simulink model "UPSControl"  (R2025b)
settings: Solver=VariableStepAuto  StartTime=0.0  StopTime=10  FixedStep=Ts  RelTol=1e-3
PostLoadFcn:
  | DataCenterParam;
values from neighbouring files (symbols this model uses):
  generator = struct    [GeneratorParam.m]
  lineInductance = 1e-6    (= 1e-06)    [DataCenterParam.m]    (also in GridParam.m)
  lineResistance = 1e-3    (= 0.001)    [DataCenterParam.m]    (also in GridParam.m)
  loadPower = 5e6    (= 5000000)    [DataCenterParam.m]    (also in LVRT.m; RedundancyAnalysis.m = 10000000)
  machine = struct    [GeneratorParam.m]
  powerTau = 0.005    [DataCenterParam.m]
  Ts = 5e-5    (= 5e-05)    [DataCenterParam.m]    (also in GeneratorParam.m)
  utilizationFactor = 0.45    [DataCenterParam.m]    (also in RedundancyAnalysis.m)
undefined symbols (not defined in the file or in its folder): breaker, ctLimitDelayTime, DiscIntNeverNeededParam, ee_sli_rtmsupport, gcbh, grid, rack, ups
libraries: nesl_utility x96, fl_lib x96, eeGeneralControl x84, ee_lib x80, simulink x68, eeTransforms x30, nesl_utility_internal x16, eeSinusoidalMeasurementV2 x13, slpidlib x12, simulink_extras x12, datacenter_lib x5, batteryecm_lib x4
(part 1 of 13)
settings Model: SimulationMode=accelerator  Creator=skota  LastModifiedBy=vikrants
settings SolverCC: ZeroCrossAlgorithm=Adaptive
settings DataIOCC: SaveOutput=off  DSMLogging=off  StreamToWks=off  SaveTime=off  ReturnWorkspaceOutputs=off
settings SimscapeCC: SimscapeCompileComponentReuse=on

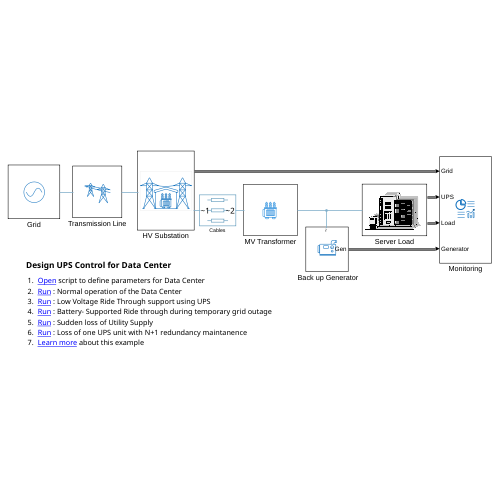
[thumbnail: Simulink's stored preview of the top-level diagram]
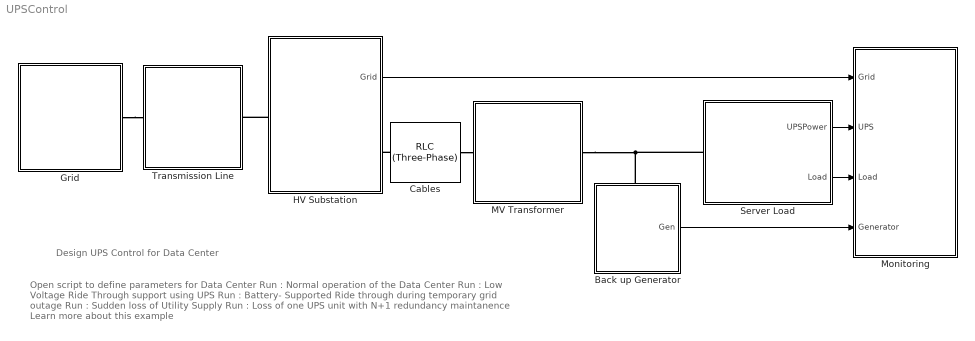
== system UPSControl ==
  note: Design UPS Control for Data Center
  note: Open script to define parameters for Data Center
      | Run : Normal operation of the Data Center
      | Run : Low Voltage Ride Through support using UPS
      | Run : Battery- Supported Ride through during temporary grid outage
      | Run : Sudden loss of Utility Supply
      | Run : Loss of one UPS unit with N+1 redundancy maintanence
      | Learn more about this example
  " Back up Generator" : Subsystem
      settings: PortSchema="{\"entries\":[{\"content\":{\"sides\":[{\"content\":{},\"type\":\"ConnectorPlacement.EquallySpacedRectSide\",\"uuid\":\"0e4bb094-5f01-4715-b678-e6b326bbface\"},{\"content\":{\"connectorIds\":[\"Out1\"],\"side\":\"RIGHT\"},\"type\":\"ConnectorPlacement.EquallySpacedRectSide\",\"uuid\":\"0cb60177-20db-48f9-a9cc-070daf12251a\"},{\"content\":{\"connectorIds\":[\"LConn1\"],\"side\":\"TOP\"},\"type\":\"ConnectorPlacement.EquallySpacedRectSide\",\"uuid\":\"205cef4a-01a9-469e-ade5-58cd4fb704d4\"},{\"content\":{\"side\":\"BOTTOM\"},\"type\":\"ConnectorPlacement.EquallySpacedRectSide\",\"uuid\":\"006e0ade-b558-4494-a2f0-eb5d5c15551c\"}]},\"type\":\"ConnectorPlacement.EquallySpacedConnector\",\"uuid\":\"9a4799c2-8742-4ae9-b78d-c2acced826f3\"}],\"packageUris\":[\"http://schema.mathworks.com/mf0/Connector/R2020b\"],\"version\":\"1.0\"}"
  Cables : ee_lib/Passive/RLC Assemblies/RLC (Three-Phase)  port_option=ee.enum.threePhasePort.composite  component_structure=ee.enum.rlc.structure.SeriesRL  R=lineResistance Ohm  L=lineInductance H  C=1e-6 F  R_parasitic=0 Ohm  G_parasitic=0 1/Ohm  IL_specify=on  IL_priority=None  IL=[0, 0, 0] A  IL_nominal_specify=off  IL_nominal_value=1  IL_nominal_unit=A  VC_specify=off  VC_priority=High  VC=[0, 0, 0] V  VC_nominal_specify=off  VC_nominal_value=1  VC_nominal_unit=V
      settings: InternalSimscapePortConfiguration="{\"Bottom\":[],\"Left\":[{\"id\":\"N1\",\"label\":\"~1\",\"type\":\"foundation.electrical.three_phase\"}],\"Right\":[{\"id\":\"N2\",\"label\":\"~2\",\"type\":\"foundation.electrical.three_phase\"}],\"Top\":[]}"
  Grid : Subsystem
  HV Substation : Subsystem
  MV Transformer : Subsystem
  Monitoring : Subsystem
  Server Load : Subsystem
      mask Display: image('datacenter.png');
  Transmission Line : Subsystem
  wires:
  Server Load/1(UPSPower) -> Monitoring/2(UPS)
  HV Substation/1(Grid) -> Monitoring/1(Grid)
  " Back up Generator"/1(Gen) -> Monitoring/4(Generator)
  Server Load/2(Load) -> Monitoring/3(Load)
  connections:
  Cables/LConn1 -- HV Substation/RConn1
  Cables/RConn1 -- MV Transformer/LConn1
  MV Transformer/RConn1 -- Server Load/LConn1 -- " Back up Generator"/LConn1
  HV Substation/LConn1 -- Transmission Line/LConn1
  Grid/LConn1 -- Transmission Line/RConn1

== system UPSControl/ Back up Generator ==
  note: Circuit breaker
  Brk Signal : Step  Time=breaker.generator  Before=1  After=0  SampleTime=0
  Cables : ee_lib/Passive/RLC Assemblies/RLC (Three-Phase)  port_option=ee.enum.threePhasePort.composite  component_structure=ee.enum.rlc.structure.SeriesRL  R=1e-3 Ohm  L=1e-5 H  C=1e-6 F  R_parasitic=0 Ohm  G_parasitic=0 1/Ohm  IL_specify=on  IL_priority=None  IL=[0, 0, 0] A  IL_nominal_specify=off  IL_nominal_value=1  IL_nominal_unit=A  VC_specify=off  VC_priority=High  VC=[0, 0, 0] V  VC_nominal_specify=off  VC_nominal_value=1  VC_nominal_unit=V
      settings: InternalSimscapePortConfiguration="{\"Bottom\":[],\"Left\":[{\"id\":\"N1\",\"label\":\"~1\",\"type\":\"foundation.electrical.three_phase\"}],\"Right\":[{\"id\":\"N2\",\"label\":\"~2\",\"type\":\"foundation.electrical.three_phase\"}],\"Top\":[]}"
  Constant : Constant  Value=0
  Generator Set : Subsystem  Variant=on  VariantControlMode=label  LabelModeActiveChoice=Detailed  mask(Generator){fidelity=Detailed, genRating=generator.rating, Vac=generator.Vac, frequency=generator.frequency, polePairs=generator.polePairs, pu_speed_reference=machine.speedReference, droop_percentage=machine.droop, pu_load_reference_setpoint=machine.loadReference, T_G=machine.timeConstandGovernor, T_CH=machine.timeConstantPrimeMover, base_torque=machine.baseTorque, pu_torque0=machine.initialTorque}
      mask prompts: fidelity "Modeling Option"; genRating "Generator Rating (kW)"; Vac "Rated AC side voltage (phase-phase RMS) (V)"; frequency "Rated electrical frequency at AC side (Hz)"; polePairs "Number of pole pairs"; pu_speed_reference "Speed reference, (pu)"; droop_percentage "Percentage droop, (%)"; pu_load_reference_setpoint "Load reference setpoint, (pu)"; T_G "Time constant of governor, (s)"; T_CH "Time constant of main inlet volumes and steam chest, (s)"; base_torque "Base torque, (N*m)"; pu_torque0 "Initial torque, (pu)"
      mask help:
      | This block models a Generator. The detailed variant models AVR, Exciter, Prime mover, and Governer. The simplified variant is based on load torque and a constant field circuit current. Select simplified mode for faster simulation using fixed efficiency and rated power.
      |
      | Provide load reference as input
      settings: CopyFcn=set_param(gcbh,'LinkStatus','none');
      mask TypeOptions fidelity: Detailed | Simplified
      mask Callback fidelity:
      | detailedTabs = {'generatorDetailed','exciterParam','governerParam',};
      |     simplifiedTabs = {'generatorSimplified'};
      |     component.mask.fidelitySelection(detailedTabs,simplifiedTabs);
      |     component.mask.fidelitySelection;
      mask TypeOptions pu_speed_reference:
      | Detailed/Governor and
      | Prime Mover
      | /pu_speed_reference
      mask TypeOptions droop_percentage:
      | Detailed/Governor and
      | Prime Mover
      | /droop_percentage
      mask TypeOptions pu_load_reference_setpoint:
      | Detailed/Governor and
      | Prime Mover
      | /pu_load_reference_setpoint
      mask TypeOptions T_G:
      | Detailed/Governor and
      | Prime Mover
      | /T_G
      mask TypeOptions T_CH:
      | Detailed/Governor and
      | Prime Mover
      | /T_CH
      mask TypeOptions base_torque:
      | Detailed/Governor and
      | Prime Mover
      | /base_torque
      mask TypeOptions pu_torque0:
      | Detailed/Governor and
      | Prime Mover
      | /pu_torque0
      mask DialogControl generalDetailed Prompt: General
      mask DialogControl editMachine Prompt: Edit machine parameters
      mask DialogControl editMachine Callback:
      | blockFidelity = get_param(gcb,'fidelity');
      |     blockPath = [gcb,'/',blockFidelity,'/','Machine'];
      |     component.mask.openBlock(blockPath);
      mask DialogControl editInertia Prompt: Edit inertia parameters
      mask DialogControl editInertia Callback:
      | blockPath = [gcb,'/','Detailed','/','Inertia'];
      |     component.mask.openBlock(blockPath);
      mask DialogControl exciterParam Prompt: Exciter
      mask DialogControl fieldParam Prompt: Edit field circuit parameters
      mask DialogControl fieldParam Callback:
      | blockPath = [gcb,'/','Detailed','/','AVR and Exciter','/','Exciter'];
      |     component.mask.openBlock(blockPath);
      mask DialogControl avrParam Prompt: Edit AVR parameters
      mask DialogControl avrParam Callback:
      | blockPath = [gcb,'/','Detailed','/','AVR and Exciter','/','AVR'];
      |     component.mask.openBlock(blockPath);
      mask DialogControl governerParam Prompt: Governer and Prime Mover
  Phase Splitter : ee_lib/Connectors & References/Phase Splitter
  Phase Splitter1 : ee_lib/Connectors & References/Phase Splitter
  Power Measurement : Subsystem
      settings: PortSchema="{\"entries\":[{\"content\":{\"sides\":[{\"content\":{\"connectorIds\":[\"LConn1\"]},\"type\":\"ConnectorPlacement.EquallySpacedRectSide\",\"uuid\":\"0c8863a2-a78f-4a73-a820-c6aa5bdc2133\"},{\"content\":{\"connectorIds\":[\"RConn1\"],\"side\":\"RIGHT\"},\"type\":\"ConnectorPlacement.EquallySpacedRectSide\",\"uuid\":\"2028a368-e468-46fb-8c3f-9ce74e7f0a45\"},{\"content\":{\"side\":\"TOP\"},\"type\":\"ConnectorPlacement.EquallySpacedRectSide\",\"uuid\":\"1b144116-ac84-43c3-ac53-ab33c5b71658\"},{\"content\":{\"connectorIds\":[\"Out1\",\"Out2\"],\"side\":\"BOTTOM\"},\"type\":\"ConnectorPlacement.EquallySpacedRectSide\",\"uuid\":\"3e4d0e65-8f44-4e57-8d60-68941db834c2\"}]},\"type\":\"ConnectorPlacement.EquallySpacedConnector\",\"uuid\":\"a27c8f54-ed82-4619-aed8-d6cf5e2c28e1\"}],\"packageUris\":[\"http://schema.mathworks.com/mf0/Connector/R2020b\"],\"version\":\"1.0\"}"
      mask Display: image('measurements.png');
  Subsystem : Subsystem
  Variable Resistor : fl_lib/Electrical/Electrical Elements/Variable Resistor  Rmin=1e-3 Ohm  thermalEnable=false  thermal_mass=1 J/K  i_specify=on  i_priority=None  i=0 A  i_nominal_specify=off  i_nominal_value=1  i_nominal_unit=A  v_specify=off  v_priority=None  v=0 V  v_nominal_specify=off  v_nominal_value=1  v_nominal_unit=V  T_specify=off  T_priority=None  T=300 K  T_nominal_specify=off  T_nominal_value=1  T_nominal_unit=K
  Variable Resistor1 : fl_lib/Electrical/Electrical Elements/Variable Resistor  Rmin=1e-3 Ohm  thermalEnable=false  thermal_mass=1 J/K  i_specify=on  i_priority=None  i=0 A  i_nominal_specify=off  i_nominal_value=1  i_nominal_unit=A  v_specify=off  v_priority=None  v=0 V  v_nominal_specify=off  v_nominal_value=1  v_nominal_unit=V  T_specify=off  T_priority=None  T=300 K  T_nominal_specify=off  T_nominal_value=1  T_nominal_unit=K
  Variable Resistor2 : fl_lib/Electrical/Electrical Elements/Variable Resistor  Rmin=1e-3 Ohm  thermalEnable=false  thermal_mass=1 J/K  i_specify=on  i_priority=None  i=0 A  i_nominal_specify=off  i_nominal_value=1  i_nominal_unit=A  v_specify=off  v_priority=None  v=0 V  v_nominal_specify=off  v_nominal_value=1  v_nominal_unit=V  T_specify=off  T_priority=None  T=300 K  T_nominal_specify=off  T_nominal_value=1  T_nominal_unit=K
  ~ : PMIOPort  Side=Left
  Bus Element Out : Outport  PortName=Gen  Element=Q
  BusElementOut : Outport  PortName=Gen  Element=P
  wires:
  Constant/1 -> Generator Set/1(PRef)
  Power Measurement/2(Q) -> Bus Element Out/1
  Power Measurement/1(P) -> BusElementOut/1
  Brk Signal/1 -> Subsystem/1(" ")
  connections:
  Generator Set/RConn1 -- Cables/LConn1
  Power Measurement/LConn1 -- Cables/RConn1
  Phase Splitter/LConn1 -- Power Measurement/RConn1
  Phase Splitter1/LConn1 -- ~/RConn1
  Variable Resistor2/LConn1 -- Variable Resistor1/LConn1 -- Variable Resistor/LConn1 -- Subsystem/RConn1
  Phase Splitter1/RConn1 -- Variable Resistor/RConn1
  Variable Resistor2/LConn2 -- Phase Splitter/RConn3
  Phase Splitter/RConn1 -- Variable Resistor/LConn2
  Phase Splitter1/RConn3 -- Variable Resistor2/RConn1
  Variable Resistor1/LConn2 -- Phase Splitter/RConn2
  Phase Splitter1/RConn2 -- Variable Resistor1/RConn1

== system UPSControl/Grid ==
  Controlled Voltage Source (Three-Phase) : ee_lib/Sources/Controlled Voltage Source (Three-Phase)  input_option=ee.enum.inputType.singleFreqAC  FRated=60 Hz
      settings: InternalSimscapePortConfiguration="{\"Bottom\":[],\"Left\":[{\"id\":\"Vt\",\"label\":\"Vt\",\"type\":\"input\"},{\"id\":\"ph\",\"label\":\"ph\",\"type\":\"input\"},{\"id\":\"n\",\"label\":\"n\",\"type\":\"foundation.electrical.electrical\"}],\"Right\":[{\"id\":\"N\",\"label\":\"~\",\"type\":\"foundation.electrical.three_phase\"}],\"Top\":[]}"
  Electrical Reference : fl_lib/Electrical/Electrical Elements/Electrical Reference
  Gain : Gain  Gain=grid.voltage
  LVRT Profile : FromWorkspace  VariableName=lvrtProfile  SampleTime=Ts  OutputAfterFinalValue=Holding final value
  PS Constant1 : fl_lib/Physical Signals/Sources/PS Constant  constant=0
  Simulink-PS Converter : nesl_utility/Simulink-PS Converter  PhysicalDomain=network_engine_domain  SubClassName=ps_input  LeftPortType=input  RightPortType=output  PseudoPeriodic=off  Frequencies=[]  NoiseDistribution=none  NoiseParameters=[]  Unit=1  AffineConversion=off  FilteringAndDerivatives=provide  SimscapeFilterOrder=1  InputFilterTimeConstant=0.001  UdotUserProvided=0
  Solver Configuration : nesl_utility/Solver Configuration  PhysicalDomain=network_engine_domain  SubClassName=solver  LeftPortType=input  RightPortType=generic  Tones=[]  Harmonics=[]  SimulateNoise=off  Profile=off  UseLocalSampling=off  EnableSwitchedLinearOptims=on  FrequencyDomain=off  UseCCode=off  RelTol=0.001  AbsTol=0.001  MinStep=1e-09  ToWorkspace=off  RevertToSquareIcSolve=off  NumHomotopyIterations=100  PhasorMode=off  PhasorModeNumHarmonics=1  ConsistencySolver=NEWTON_XTOL_AFTER_FTOL  IndexReductionMethod=None  DoDC=off  ResidualTolerance=1e-09  ConsistencyTolSource=GLOBAL  ConsistencyAbsTol=0.001  ConsistencyRelTol=0.001  ConsistencyTolFactor=1e3  UseLocalSolver=on  LocalSolverChoice=NE_BACKWARD_EULER_ADVANCER  ResolveIndetEquations=off  FunctionEvalNumThread=1  LocalSolverSampleTime=5e-05  DoFixedCost=on  MaxNonlinIter=1  MaxModeIter=2  ComputeImpulses=off  ImpulseIterations=2  LinearAlgebra=auto  LinearAlgebraNumThread=0  EquationFormulation=NE_TIME_EF  DelaysMemoryBudget=1024  AutomaticFiltering=off  FilteringTimeConstant=0.001  PartitionStorageMethod=AS_NEEDED  PartitionMemoryBudget=1024  PartitionMethod=ROBUST  MultibodyUseLocalSolver=off  MultibodyLocalSolverChoice=ODE1  MultibodyLocalSolverSampleTime=0.001
  " " : PMIOPort  Side=Left
  wires:
  LVRT Profile/1 -> Gain/1
  Gain/1 -> Simulink-PS Converter/1
  connections:
  Controlled Voltage Source (Three-Phase)/LConn3 -- Electrical Reference/LConn1
  Controlled Voltage Source (Three-Phase)/RConn1 -- " "/RConn1 -- Solver Configuration/RConn1
  PS Constant1/RConn1 -- Controlled Voltage Source (Three-Phase)/LConn2
  Controlled Voltage Source (Three-Phase)/LConn1 -- Simulink-PS Converter/RConn1

== system UPSControl/HV Substation ==
  Circuit Breaker : Subsystem
  Gain : Gain  Gain=1/(sqrt(2)*grid.voltage)
  Line Voltage Sensor (Three-Phase) : ee_lib/Sensors & Transducers/Line Voltage Sensor (Three-Phase)
  PS-Simulink Converter : nesl_utility/PS-Simulink Converter  PhysicalDomain=network_engine_domain  SubClassName=ps_output  LeftPortType=input  RightPortType=output  PseudoPeriodic=off  Frequencies=[]  VectorFormat=inherit  Unit=inherit  AffineConversion=off
  Power Measurement : Subsystem
      settings: PortSchema="{\"entries\":[{\"content\":{\"sides\":[{\"content\":{\"connectorIds\":[\"LConn1\"]},\"type\":\"ConnectorPlacement.EquallySpacedRectSide\",\"uuid\":\"0c8863a2-a78f-4a73-a820-c6aa5bdc2133\"},{\"content\":{\"connectorIds\":[\"RConn1\"],\"side\":\"RIGHT\"},\"type\":\"ConnectorPlacement.EquallySpacedRectSide\",\"uuid\":\"2028a368-e468-46fb-8c3f-9ce74e7f0a45\"},{\"content\":{\"side\":\"TOP\"},\"type\":\"ConnectorPlacement.EquallySpacedRectSide\",\"uuid\":\"1b144116-ac84-43c3-ac53-ab33c5b71658\"},{\"content\":{\"connectorIds\":[\"Out1\",\"Out2\"],\"side\":\"BOTTOM\"},\"type\":\"ConnectorPlacement.EquallySpacedRectSide\",\"uuid\":\"3e4d0e65-8f44-4e57-8d60-68941db834c2\"}]},\"type\":\"ConnectorPlacement.EquallySpacedConnector\",\"uuid\":\"a27c8f54-ed82-4619-aed8-d6cf5e2c28e1\"}],\"packageUris\":[\"http://schema.mathworks.com/mf0/Connector/R2020b\"],\"version\":\"1.0\"}"
      mask Display: image('measurements.png');
  Step : Step  Time=breaker.grid  SampleTime=0
  Terminator : Terminator
  Transformer : Subsystem  Variant=on  VariantControlMode=label  LabelModeActiveChoice=Detailed  mask{fidelity=Detailed}
      mask prompts: fidelity "Modeling Option"
      mask TypeOptions fidelity: Detailed | Simplified
      mask Callback fidelity:
      | choice = get_param(gcb,'fidelity');
      | switch choice
      |     case 'Detailed'
      |         set_param(gcb, 'LabelModeActiveChoice', 'Detailed');
      |     case 'Simplified'
      |          set_param(gcb, 'LabelModeActiveChoice', 'Simplified');
      |     otherwise
      |         disp('Choose proper variant');
      | end
  Conn1 : PMIOPort  Side=Left
  ~ : PMIOPort  Port=2  Side=Right
  Bus Element Out : Outport  PortName=Grid  Element=P
  BusElementOut : Outport  PortName=Grid  Element=Q
  wires:
  Power Measurement/1(Q) -> BusElementOut/1  "Grid"
  Power Measurement/2(P) -> Bus Element Out/1  "Grid"
  Step/1 -> Circuit Breaker/1(BRK)
  PS-Simulink Converter/1 -> Gain/1
  Gain/1 -> Terminator/1
  connections:
  Power Measurement/RConn1 -- Line Voltage Sensor (Three-Phase)/LConn1 -- Transformer/LConn1
  Power Measurement/LConn1 -- Conn1/RConn1
  Circuit Breaker/LConn1 -- Transformer/RConn1
  ~/RConn1 -- Circuit Breaker/RConn1
  Line Voltage Sensor (Three-Phase)/RConn1 -- PS-Simulink Converter/LConn1

== system UPSControl/MV Transformer ==
  Transformer : Subsystem  Variant=on  VariantControlMode=label  LabelModeActiveChoice=Detailed  mask{fidelity=Detailed}
      mask prompts: fidelity "Modeling Option"
      mask TypeOptions fidelity: Detailed | Simplified
      mask Callback fidelity:
      | choice = get_param(gcb,'fidelity');
      | switch choice
      |     case 'Detailed'
      |         set_param(gcb, 'LabelModeActiveChoice', 'Detailed');
      |     case 'Simplified'
      |          set_param(gcb, 'LabelModeActiveChoice', 'Simplified');
      |     otherwise
      |         disp('Choose proper variant');
      | end
  " " : PMIOPort  Side=Left
  "  " : PMIOPort  Port=2  Side=Right
  connections:
  Transformer/RConn1 -- "  "/RConn1
  " "/RConn1 -- Transformer/LConn1

== system UPSControl/Monitoring ==
  Bus Element In : Inport  PortName=Grid  Element=P
  BusElementIn : Inport  PortName=Grid  Element=Q
  Bus Element In3 : Inport  Port=2  PortName=UPS  Element=P
  BusElementIn2 : Inport  Port=2  PortName=UPS  Element=Q
  Bus Element In5 : Inport  Port=3  PortName=Load  Element=P
  BusElementIn5 : Inport  Port=3  PortName=Load  Element=Q
  Bus Element In4 : Inport  Port=4  PortName=Generator  Element=P
  BusElementIn4 : Inport  Port=4  PortName=Generator  Element=Q
  Mux : Mux
  Mux1 : Mux
  Power : Scope
      settings: ActiveDisplayYMinimum=-2.1915485451701304  ActiveDisplayYMaximum=14.338676802213223  YLabel=Active Power (MW)  DataLoggingVariableName=ScopeData11
  Reactive Power : Scope
      settings: ActiveDisplayYMinimum=-1.8163883606898998  ActiveDisplayYMaximum=0.79015946510747415  YLabel=Active Power (MW)  DataLoggingVariableName=ScopeData31
  wires:
  Bus Element In/1 -> Mux/1  "Grid"
  Mux/1 -> Power/1
  BusElementIn/1 -> Mux1/1  "Grid"
  Mux1/1 -> Reactive Power/1
  Bus Element In5/1 -> Mux/4  "Load"
  Bus Element In4/1 -> Mux/3  "Generator"
  Bus Element In3/1 -> Mux/2  "UPS"
  BusElementIn2/1 -> Mux1/2  "UPS"
  BusElementIn4/1 -> Mux1/3  "Generator"
  BusElementIn5/1 -> Mux1/4  "Load"

== system UPSControl/Server Load ==
  Charging Current : Constant  Value=0
  Measurements : Subsystem
  Server Racks : Subsystem
  Signal Logging : Subsystem
  UPS Units : Subsystem  Variant=on  mask{upsConfiguration=Three UPS Parallel}
      mask prompts: upsConfiguration "UPS Configuration"
      mask init:
      | val = get_param(gcb, 'upsConfiguration');
      | switch val
      |     case 'Single UPS'
      |         assignin('base', 'upsConfig', 1);
      |     case 'Three UPS Parallel'
      |         assignin('base', 'upsConfig', 3);
      | end
      mask TypeOptions upsConfiguration: Single UPS | Three UPS Parallel
      mask Callback upsConfiguration:
      | val = get_param(gcb, 'upsConfiguration');
      | switch val
      |     case 'Single UPS'
      |         assignin('base', 'upsConfig', 1);
      |     case 'Three UPS Parallel'
      |         assignin('base', 'upsConfig', 3);
      | end
      mask Display: disp('UPS Units')
  Connection Port : PMIOPort  Side=Left
  Bus Element Out1 : Outport  PortName=UPSPower  Element=P
  BusElementOut1 : Outport  PortName=UPSPower  Element=Q
  Bus Element Out : Outport  Port=2  PortName=Load  Element=P
  BusElementOut : Outport  Port=2  PortName=Load  Element=Q
  wires:
  Charging Current/1 -> UPS Units/1(iChrg)
  Measurements/2(Q) -> BusElementOut/1
  Measurements/1(P) -> Bus Element Out/1
  UPS Units/1(Meas) -> Signal Logging/1(Meas)
  UPS Units/2(P) -> Bus Element Out1/1
  UPS Units/3(Q) -> BusElementOut1/1
  connections:
  Connection Port/RConn1 -- UPS Units/LConn1
  Measurements/LConn1 -- UPS Units/RConn1
  Server Racks/LConn1 -- Measurements/RConn1

== system UPSControl/Transmission Line ==
  RLC (Three-Phase) : ee_lib/Passive/RLC Assemblies/RLC (Three-Phase)  port_option=ee.enum.threePhasePort.composite  component_structure=ee.enum.rlc.structure.SeriesRL  R=1e-2*10 Ohm  L=1e-6*10 H  C=1e-6 F  R_parasitic=0 Ohm  G_parasitic=0 1/Ohm  IL_specify=on  IL_priority=None  IL=[0, 0, 0] A  IL_nominal_specify=off  IL_nominal_value=1  IL_nominal_unit=A  VC_specify=off  VC_priority=High  VC=[0, 0, 0] V  VC_nominal_specify=off  VC_nominal_value=1  VC_nominal_unit=V
      settings: InternalSimscapePortConfiguration="{\"Bottom\":[],\"Left\":[{\"id\":\"N1\",\"label\":\"~1\",\"type\":\"foundation.electrical.three_phase\"}],\"Right\":[{\"id\":\"N2\",\"label\":\"~2\",\"type\":\"foundation.electrical.three_phase\"}],\"Top\":[]}"
  Out : PMIOPort  Side=Left
  In : PMIOPort  Port=2  Side=Right
  connections:
  RLC (Three-Phase)/LConn1 -- In/RConn1
  RLC (Three-Phase)/RConn1 -- Out/RConn1

== system UPSControl/ Back up Generator/Generator Set ==
  PRef : Inport
  Detailed : Subsystem  VariantControl=Detailed
  Simplified : Subsystem  VariantControl=Simplified
  ~ : PMIOPort  Side=Right
  Meas : Outport

== system UPSControl/ Back up Generator/Power Measurement ==
  Low-Pass Filter (Discrete or Continuous) : eeGeneralControl/Low-Pass Filter (Discrete or Continuous)  K=1  T=powerTau  B=inf  A=-inf  init_option=Inherited from block input  x0=0  Ts=-1
  Low-Pass Filter (Discrete or Continuous)1 : eeGeneralControl/Low-Pass Filter (Discrete or Continuous)  K=1  T=powerTau  B=inf  A=-inf  init_option=Inherited from block input  x0=0  Ts=-1
  PS-Simulink Converter2 : nesl_utility/PS-Simulink Converter  PhysicalDomain=network_engine_domain  SubClassName=ps_output  LeftPortType=input  RightPortType=output  PseudoPeriodic=off  Frequencies=[]  VectorFormat=inherit  Unit=MW  AffineConversion=off
  PS-Simulink Converter3 : nesl_utility/PS-Simulink Converter  PhysicalDomain=network_engine_domain  SubClassName=ps_output  LeftPortType=input  RightPortType=output  PseudoPeriodic=off  Frequencies=[]  VectorFormat=inherit  Unit=MW  AffineConversion=off
  Power Sensor (Three-Phase) : ee_lib/Sensors & Transducers/Power Sensor (Three-Phase)  load_type=ee.enum.passive.type_balanced.balanced  f0=60 Hz
      settings: InternalSimscapePortConfiguration="{\"Bottom\":[],\"Left\":[{\"id\":\"N1\",\"label\":\"~1\",\"type\":\"foundation.electrical.three_phase\"}],\"Right\":[{\"id\":\"N2\",\"label\":\"~2\",\"type\":\"foundation.electrical.three_phase\"}],\"Top\":[{\"id\":\"Pm\",\"label\":\"P\",\"type\":\"output\"},{\"id\":\"Qm\",\"label\":\"Q\",\"type\":\"output\"}]}"
  Scope1 : Scope  NumInputPorts=2
      settings: ActiveDisplayYMinimum=-1  ActiveDisplayYMaximum=1  DataLoggingVariableName=ScopeData2
  In : PMIOPort  Side=Left
  Out : PMIOPort  Port=2  Side=Right
  P : Outport
  Q : Outport  Port=2
  wires:
  PS-Simulink Converter3/1 -> Low-Pass Filter (Discrete or Continuous)1/1, Scope1/2
  PS-Simulink Converter2/1 -> Low-Pass Filter (Discrete or Continuous)/1, Scope1/1
  Low-Pass Filter (Discrete or Continuous)/1 -> P/1
  Low-Pass Filter (Discrete or Continuous)1/1 -> Q/1
  connections:
  Power Sensor (Three-Phase)/RConn1 -- Out/RConn1
  PS-Simulink Converter2/LConn1 -- Power Sensor (Three-Phase)/LConn2
  PS-Simulink Converter3/LConn1 -- Power Sensor (Three-Phase)/LConn3
  Power Sensor (Three-Phase)/LConn1 -- In/RConn1

== system UPSControl/ Back up Generator/Subsystem ==
  " " : Inport
  Data Type Conversion : DataTypeConversion  OutDataTypeStr=double  SaturateOnIntegerOverflow=off  RndMeth=Floor
  Open Resistance : Gain  Gain=5e6
  Simulink-PS Converter : nesl_utility/Simulink-PS Converter  PhysicalDomain=network_engine_domain  SubClassName=ps_input  LeftPortType=input  RightPortType=output  PseudoPeriodic=off  Frequencies=[]  NoiseDistribution=none  NoiseParameters=[]  Unit=1  AffineConversion=off  FilteringAndDerivatives=provide  SimscapeFilterOrder=1  InputFilterTimeConstant=0.001  UdotUserProvided=0
  "  " : PMIOPort  Side=Right
  wires:
  Data Type Conversion/1 -> Open Resistance/1
  Open Resistance/1 -> Simulink-PS Converter/1
  " "/1 -> Data Type Conversion/1
  connections:
  Simulink-PS Converter/RConn1 -- "  "/RConn1

== system UPSControl/HV Substation/Circuit Breaker ==
  BRK : Inport
  Data Type Conversion : DataTypeConversion  OutDataTypeStr=double  SaturateOnIntegerOverflow=off  RndMeth=Floor
  Open Resistance : Gain  Gain=5e6
  Phase Splitter : ee_lib/Connectors & References/Phase Splitter
  Phase Splitter1 : ee_lib/Connectors & References/Phase Splitter
  Simulink-PS Converter : nesl_utility/Simulink-PS Converter  PhysicalDomain=network_engine_domain  SubClassName=ps_input  LeftPortType=input  RightPortType=output  PseudoPeriodic=off  Frequencies=[]  NoiseDistribution=none  NoiseParameters=[]  Unit=1  AffineConversion=off  FilteringAndDerivatives=provide  SimscapeFilterOrder=1  InputFilterTimeConstant=0.001  UdotUserProvided=0
  Variable Resistor : fl_lib/Electrical/Electrical Elements/Variable Resistor  Rmin=1e-3 Ohm  thermalEnable=false  thermal_mass=1 J/K  i_specify=on  i_priority=None  i=0 A  i_nominal_specify=off  i_nominal_value=1  i_nominal_unit=A  v_specify=off  v_priority=None  v=0 V  v_nominal_specify=off  v_nominal_value=1  v_nominal_unit=V  T_specify=off  T_priority=None  T=300 K  T_nominal_specify=off  T_nominal_value=1  T_nominal_unit=K
  Variable Resistor1 : fl_lib/Electrical/Electrical Elements/Variable Resistor  Rmin=1e-3 Ohm  thermalEnable=false  thermal_mass=1 J/K  i_specify=on  i_priority=None  i=0 A  i_nominal_specify=off  i_nominal_value=1  i_nominal_unit=A  v_specify=off  v_priority=None  v=0 V  v_nominal_specify=off  v_nominal_value=1  v_nominal_unit=V  T_specify=off  T_priority=None  T=300 K  T_nominal_specify=off  T_nominal_value=1  T_nominal_unit=K
  Variable Resistor2 : fl_lib/Electrical/Electrical Elements/Variable Resistor  Rmin=1e-3 Ohm  thermalEnable=false  thermal_mass=1 J/K  i_specify=on  i_priority=None  i=0 A  i_nominal_specify=off  i_nominal_value=1  i_nominal_unit=A  v_specify=off  v_priority=None  v=0 V  v_nominal_specify=off  v_nominal_value=1  v_nominal_unit=V  T_specify=off  T_priority=None  T=300 K  T_nominal_specify=off  T_nominal_value=1  T_nominal_unit=K
  In : PMIOPort  Side=Left
  ~ : PMIOPort  Port=2  Side=Right
  wires:
  Data Type Conversion/1 -> Open Resistance/1
  BRK/1 -> Data Type Conversion/1
  Open Resistance/1 -> Simulink-PS Converter/1
  connections:
  Phase Splitter1/RConn2 -- Variable Resistor1/RConn1
  Variable Resistor1/LConn2 -- Phase Splitter/RConn2
  Phase Splitter1/RConn3 -- Variable Resistor2/RConn1
  Phase Splitter/RConn1 -- Variable Resistor/LConn2
  Variable Resistor2/LConn2 -- Phase Splitter/RConn3
  Phase Splitter1/RConn1 -- Variable Resistor/RConn1
  Phase Splitter1/LConn1 -- ~/RConn1
  Variable Resistor/LConn1 -- Simulink-PS Converter/RConn1 -- Variable Resistor2/LConn1 -- Variable Resistor1/LConn1
  Phase Splitter/LConn1 -- In/RConn1

== system UPSControl/HV Substation/Power Measurement ==
  Low-Pass Filter (Discrete or Continuous) : eeGeneralControl/Low-Pass Filter (Discrete or Continuous)  K=1  T=powerTau  B=inf  A=-inf  init_option=Inherited from block input  x0=0  Ts=-1
  Low-Pass Filter (Discrete or Continuous)1 : eeGeneralControl/Low-Pass Filter (Discrete or Continuous)  K=1  T=powerTau  B=inf  A=-inf  init_option=Inherited from block input  x0=0  Ts=-1
  PS-Simulink Converter2 : nesl_utility/PS-Simulink Converter  PhysicalDomain=network_engine_domain  SubClassName=ps_output  LeftPortType=input  RightPortType=output  PseudoPeriodic=off  Frequencies=[]  VectorFormat=inherit  Unit=MW  AffineConversion=off
  PS-Simulink Converter3 : nesl_utility/PS-Simulink Converter  PhysicalDomain=network_engine_domain  SubClassName=ps_output  LeftPortType=input  RightPortType=output  PseudoPeriodic=off  Frequencies=[]  VectorFormat=inherit  Unit=MW  AffineConversion=off
  Power Sensor (Three-Phase) : ee_lib/Sensors & Transducers/Power Sensor (Three-Phase)  load_type=ee.enum.passive.type_balanced.balanced  f0=60 Hz
      settings: InternalSimscapePortConfiguration="{\"Bottom\":[],\"Left\":[{\"id\":\"N1\",\"label\":\"~1\",\"type\":\"foundation.electrical.three_phase\"}],\"Right\":[{\"id\":\"N2\",\"label\":\"~2\",\"type\":\"foundation.electrical.three_phase\"}],\"Top\":[{\"id\":\"Pm\",\"label\":\"P\",\"type\":\"output\"},{\"id\":\"Qm\",\"label\":\"Q\",\"type\":\"output\"}]}"
  In : PMIOPort  Side=Left
  Out : PMIOPort  Port=2  Side=Right
  Q : Outport
  P : Outport  Port=2
  wires:
  PS-Simulink Converter2/1 -> Low-Pass Filter (Discrete or Continuous)/1
  Low-Pass Filter (Discrete or Continuous)/1 -> P/1
  PS-Simulink Converter3/1 -> Low-Pass Filter (Discrete or Continuous)1/1
  Low-Pass Filter (Discrete or Continuous)1/1 -> Q/1
  connections:
  Power Sensor (Three-Phase)/LConn1 -- In/RConn1
  Power Sensor (Three-Phase)/RConn1 -- Out/RConn1
  PS-Simulink Converter2/LConn1 -- Power Sensor (Three-Phase)/LConn2
  PS-Simulink Converter3/LConn1 -- Power Sensor (Three-Phase)/LConn3

== system UPSControl/HV Substation/Transformer ==
  Detailed : Subsystem  VariantControl=Detailed
  Simplified : Subsystem  VariantControl=Simplified  mask{windingRatio=13500/6600}
      mask prompts: windingRatio "Winding ratio"
      mask DialogControl Container4 Prompt: General
  In : PMIOPort  Side=Left
  Out : PMIOPort  Port=2  Side=Right

== system UPSControl/MV Transformer/Transformer ==
  Detailed : Subsystem  VariantControl=Detailed
  Simplified : Subsystem  VariantControl=Simplified  mask{windingRatio=13500/6600}
      mask prompts: windingRatio "Winding ratio"
      mask DialogControl Container4 Prompt: General
  In : PMIOPort  Side=Left
  Out : PMIOPort  Port=2  Side=Right

== system UPSControl/Server Load/Measurements ==
  Current and Voltage Sensor (Three-Phase)1 : ee_lib/Sensors & Transducers/Current and Voltage Sensor (Three-Phase)  vMeasurementType=ee.enum.vmeasurement.ll  outputUnit=ee.enum.unit.pu  SRated=loadPower A*V  VRated=ups.Vac V  I_specify=off  I_priority=None  I=[0, 0, 0] A  I_nominal_specify=off  I_nominal_value=1  I_nominal_unit=A  V_specify=off  V_priority=None  V=[0, 0, 0] V  V_nominal_specify=off  V_nominal_value=1  V_nominal_unit=V
      settings: InternalSimscapePortConfiguration="{\"Bottom\":[],\"Left\":[{\"id\":\"N1\",\"label\":\"~1\",\"type\":\"foundation.electrical.three_phase\"}],\"Right\":[{\"id\":\"V_output\",\"label\":\"V\",\"type\":\"output\"},{\"id\":\"I_output\",\"label\":\"I\",\"type\":\"output\"},{\"id\":\"N2\",\"label\":\"~2\",\"type\":\"foundation.electrical.three_phase\"}],\"Top\":[]}"
  Gain : Gain  Gain=1/1e6
  Gain1 : Gain  Gain=1/1e6
  Gain2 : Gain  Gain=loadPower/5e6
  Low-Pass Filter (Discrete or Continuous) : eeGeneralControl/Low-Pass Filter (Discrete or Continuous)  K=1  T=powerTau  B=inf  A=-inf  init_option=Inherited from block input  x0=0  Ts=-1
  Low-Pass Filter (Discrete or Continuous)1 : eeGeneralControl/Low-Pass Filter (Discrete or Continuous)  K=1  T=powerTau  B=inf  A=-inf  init_option=Inherited from block input  x0=0  Ts=-1
  PS RMS Estimator : fl_lib/Physical Signals/Periodic Operators/PS RMS Estimator  f0=60 Hz
      settings: InternalSimscapePortConfiguration="{\"Bottom\":[],\"Left\":[{\"id\":\"I\",\"label\":\"\",\"type\":\"input\"}],\"Right\":[{\"id\":\"O\",\"label\":\"\",\"type\":\"output\"}],\"Top\":[]}"
  PS RMS Estimator1 : fl_lib/Physical Signals/Periodic Operators/PS RMS Estimator  f0=60 Hz
      settings: InternalSimscapePortConfiguration="{\"Bottom\":[],\"Left\":[{\"id\":\"I\",\"label\":\"\",\"type\":\"input\"}],\"Right\":[{\"id\":\"O\",\"label\":\"\",\"type\":\"output\"}],\"Top\":[]}"
  PS-Simulink Converter{,1..5} (6 alike) : nesl_utility/PS-Simulink Converter  PhysicalDomain=network_engine_domain  SubClassName=ps_output  LeftPortType=input  RightPortType=output  PseudoPeriodic=off  Frequencies=[]  VectorFormat=inherit  Unit=inherit  AffineConversion=off
  Power Sensor (Three-Phase) : ee_lib/Sensors & Transducers/Power Sensor (Three-Phase)  load_type=ee.enum.passive.type_balanced.balanced  f0=60 Hz
      settings: InternalSimscapePortConfiguration="{\"Bottom\":[],\"Left\":[{\"id\":\"N1\",\"label\":\"~1\",\"type\":\"foundation.electrical.three_phase\"}],\"Right\":[{\"id\":\"N2\",\"label\":\"~2\",\"type\":\"foundation.electrical.three_phase\"}],\"Top\":[{\"id\":\"Pm\",\"label\":\"P\",\"type\":\"output\"},{\"id\":\"Qm\",\"label\":\"Q\",\"type\":\"output\"}]}"
  RLC (Three-Phase) : ee_lib/Passive/RLC Assemblies/RLC (Three-Phase)  port_option=ee.enum.threePhasePort.composite  component_structure=ee.enum.rlc.structure.SeriesRL  R=1e-3%1e-4 Ohm  L=1e-6%1e-6 H  C=1e-6 F  R_parasitic=0 Ohm  G_parasitic=0 1/Ohm  IL_specify=on  IL_priority=None  IL=[0, 0, 0] A  IL_nominal_specify=off  IL_nominal_value=1  IL_nominal_unit=A  VC_specify=off  VC_priority=High  VC=[0, 0, 0] V  VC_nominal_specify=off  VC_nominal_value=1  VC_nominal_unit=V
      settings: InternalSimscapePortConfiguration="{\"Bottom\":[],\"Left\":[{\"id\":\"N1\",\"label\":\"~1\",\"type\":\"foundation.electrical.three_phase\"}],\"Right\":[{\"id\":\"N2\",\"label\":\"~2\",\"type\":\"foundation.electrical.three_phase\"}],\"Top\":[]}"
  Terminator{,1,8..9} (4 alike) : Terminator
  Conn1 : PMIOPort  Side=Left
  ~ : PMIOPort  Port=2  Side=Right
  P : Outport
  Q : Outport  Port=2
  wires:
  Gain/1 -> Low-Pass Filter (Discrete or Continuous)/1
  PS-Simulink Converter5/1 -> Terminator8/1
  PS-Simulink Converter4/1 -> Terminator9/1
  Gain1/1 -> Low-Pass Filter (Discrete or Continuous)1/1
  Gain2/1 -> Terminator1/1  "Load"
  PS-Simulink Converter3/1 -> Gain2/1
  PS-Simulink Converter/1 -> Terminator/1  "Load"
  Low-Pass Filter (Discrete or Continuous)1/1 -> Q/1  "Load"
  PS-Simulink Converter2/1 -> Gain1/1
  PS-Simulink Converter1/1 -> Gain/1
  Low-Pass Filter (Discrete or Continuous)/1 -> P/1  "Load"
  connections:
  PS-Simulink Converter3/LConn1 -- PS RMS Estimator1/LConn1 -- Current and Voltage Sensor (Three-Phase)1/RConn2
  PS-Simulink Converter/LConn1 -- PS RMS Estimator/LConn1 -- Current and Voltage Sensor (Three-Phase)1/RConn1
  Current and Voltage Sensor (Three-Phase)1/RConn3 -- ~/RConn1
  PS-Simulink Converter1/LConn1 -- Power Sensor (Three-Phase)/LConn2
  PS-Simulink Converter5/LConn1 -- PS RMS Estimator1/RConn1
  Power Sensor (Three-Phase)/RConn1 -- RLC (Three-Phase)/LConn1
  Current and Voltage Sensor (Three-Phase)1/LConn1 -- RLC (Three-Phase)/RConn1
  Conn1/RConn1 -- Power Sensor (Three-Phase)/LConn1
  PS-Simulink Converter2/LConn1 -- Power Sensor (Three-Phase)/LConn3
  PS-Simulink Converter4/LConn1 -- PS RMS Estimator/RConn1

== system UPSControl/Server Load/Server Racks ==
  Efficiency Gain : fl_lib/Physical Signals/Functions/PS Gain  gain=rack.efficiencyGain
  Gain1 : Gain  Gain=utilizationFactor
  Load : ee_lib/Passive/Dynamic Load (Three-Phase)  port_option=ee.enum.threePhasePort.composite  FRated=60 Hz  Vline_rms_min=100 V  tau=0.01 s  Vline_rms_ini=1e-4 V  Vang_ini=0 deg  gmin=1e-5 S
      settings: InternalSimscapePortConfiguration="{\"Bottom\":[],\"Left\":[{\"id\":\"N\",\"label\":\"~\",\"type\":\"foundation.electrical.three_phase\"}],\"Right\":[],\"Top\":[{\"id\":\"P\",\"label\":\"P\",\"type\":\"input\"},{\"id\":\"Q\",\"label\":\"Q\",\"type\":\"input\"}]}"
  PDU Racks : Subsystem  mask{nTrays=rack.nTrays, nRacks=rack.nRacks, trayMass=rack.trayMass, trayCp=rack.trayCp, trayThermalR=rack.trayThermalR, nGPU=rack.nGPU, gpuTDPperDie=rack.gpuTDPperDie, gpuIdlePower=rack.gpuIdlePower, gpuHBMpower=rack.gpuHBMpower, gpuExponent=rack.gpuExponent, gpuHBMutil=rack.gpuHBMutil, gpuLeakage=rack.gpuLeakage, gpuNominalDieT=rack.gpuNominalDieT, gpuDieThermalC=rack.gpuDieThermalC, gpuHeatSinkR=rack.gpuHeatSinkR, gpuSurfArea=rack.gpuSurfArea, gpuAmbientR=rack.gpuAmbientR, nCPU=rack.nCPU, cpuTDPperSocket=rack.cpuTDPperSocket, cpuIdlePower=rack.cpuIdlePower, cpuExponent=rack.cpuExponent, cpuLeakage=rack.cpuLeakage, cpuNominalDieT=rack.cpuNominalDieT, cpuDieThermalC=rack.cpuDieThermalC, cpuHeatSinkR=rack.cpuHeatSinkR, cpuSurfArea=rack.cpuSurfArea, cpuAmbientR=rack.cpuAmbientR, initialT=rack.initialT, htc=rack.htc}
      mask prompts: nTrays "Number of IT trays per rack (-)"; nRacks "Number of racks (-)"; trayMass "Tray mass (kg)"; trayCp "Tray specific heat capacity (J/kg*K)"; trayThermalR "Tray to external thermal resistance (K/W)"; nGPU "Number of GPU per tray (-)"; gpuTDPperDie "GPU TDP per die (W)"; gpuIdlePower "GPU idle power (W)"; gpuHBMpower "HBM power per GPU (W)"; gpuExponent "GPU power utilization exponent (-)"; gpuHBMutil "HBM utilization as fraction of compute utilization (-)"; gpuLeakage "Leakage increase per K above nominal temperature (W/K)"; gpuNominalDieT "Nominal die temperature at TDP (K)"; gpuDieThermalC "GPU die thermal capacitance (J/K)"; gpuHeatSinkR "GPU die-heat-sink thermal resistance (K/W)"; gpuSurfArea "Surface area per die for ambient heat transfer (m^2)"; gpuAmbientR "GPU die-ambient thermal resistance (K/W)"; nCPU "Number of CPU per tray (-)"; cpuTDPperSocket "CPU TDP per socket (W)"; cpuIdlePower "CPU idle power per socket (W)"; cpuExponent "CPU power utilization exponent (-)"; cpuLeakage "Leakage increase per K above nominal temperature (W/K)"; cpuNominalDieT "Nominal die temperature at TDP (K)"; cpuDieThermalC "CPU die thermal capacitance (J/K)"; cpuHeatSinkR "CPU die-heat-sink thermal resistance (K/W)"; cpuSurfArea "Surface area per die for ambient heat transfer (m^2)"; cpuAmbientR "CPU die-ambient thermal resistance (K/W)"; initialT "Initial temperature (K)"; htc "Heat transfer coefficient to ambient (W/m^2.K)"
      settings: CopyFcn=set_param(gcbh,'LinkStatus','none');  PortSchema="{\"entries\":[{\"content\":{\"sides\":[{\"content\":{\"connectorIds\":[\"LConn1\",\"LConn2\",\"LConn3\"]},\"type\":\"ConnectorPlacement.EquallySpacedRectSide\",\"uuid\":\"1a9a884a-dab1-4495-bf62-c6b2de6c1039\"},{\"content\":{\"connectorIds\":[\"RConn1\",\"RConn2\",\"RConn3\"],\"side\":\"RIGHT\"},\"type\":\"ConnectorPlacement.EquallySpacedRectSide\",\"uuid\":\"05c53434-51c1-4fee-b885-c321dcda8b6b\"},{\"content\":{\"side\":\"TOP\"},\"type\":\"ConnectorPlacement.EquallySpacedRectSide\",\"uuid\":\"c7b5c534-d596-4858-a133-27f005e6c9d4\"},{\"content\":{\"connectorIds\":[\"RConn4\"],\"side\":\"BOTTOM\"},\"type\":\"ConnectorPlacement.EquallySpacedRectSide\",\"uuid\":\"693f3c99-4296-4d86-bfcc-da753d3e576f\"}]},\"type\":\"ConnectorPlacement.EquallySpacedConnector\",\"uuid\":\"ed91c467-c4d0-403f-af16-bac0257594fd\"}],\"packageUris\":[\"http://schema.mathworks.com/mf0/Connector/R2020b\"],\"version\":\"1.0\"}"
      mask Help: web("DocumentationPDURacks.html")
      mask DialogControl Container10 Prompt: PDU Racks
      mask DialogControl getRatingButton Prompt: Get Rating
      mask DialogControl Container9 Prompt: IT Tray
      mask DialogControl Container6 Prompt: GPU
      mask DialogControl Container7 Prompt: CPU
      mask DialogControl Container8 Prompt: Initial Conditions
      mask Display: image('icon_PDURacks.png');
  Simulink-PS Converter : nesl_utility/Simulink-PS Converter  PhysicalDomain=network_engine_domain  SubClassName=ps_input  LeftPortType=input  RightPortType=output  PseudoPeriodic=off  Frequencies=[]  NoiseDistribution=none  NoiseParameters=[]  Unit=1  AffineConversion=off  FilteringAndDerivatives=provide  SimscapeFilterOrder=1  InputFilterTimeConstant=0.001  UdotUserProvided=0
  THD : datacenter_lib/Custom Dynamic Load (3-phase) block  Pf=1  THD=0  N=1
      settings: InternalSimscapePortConfiguration="{\"Bottom\":[],\"Left\":[{\"id\":\"Pw\",\"label\":\"Pvec\",\"type\":\"input\"}],\"Right\":[{\"id\":\"P\",\"label\":\"P\",\"type\":\"output\"},{\"id\":\"Q\",\"label\":\"Q\",\"type\":\"output\"}],\"Top\":[]}"
  TermC_Ha : fl_lib/Thermal/Thermal Elements/Thermal Mass  mass_type=foundation.enum.constant_variable.constant  mass=1e4 kg  sp_heat=1000 J/(K*kg)  mass_min=1e-6 kg  num_ports=foundation.enum.numPorts2.one  m_specify=off  m_priority=None  m=1 kg  m_nominal_specify=off  m_nominal_value=1  m_nominal_unit=kg  T_specify=off  T_priority=None  T=308.15 K  T_nominal_specify=off  T_nominal_value=1  T_nominal_unit=K  Q_specify=off  Q_priority=None  Q=0 W  Q_nominal_specify=off  Q_nominal_value=1  Q_nominal_unit=W
  TermC_Hc : fl_lib/Thermal/Thermal Elements/Thermal Mass  mass_type=foundation.enum.constant_variable.constant  mass=1e4 kg  sp_heat=1000 J/(K*kg)  mass_min=1e-6 kg  num_ports=foundation.enum.numPorts2.one  m_specify=off  m_priority=None  m=1 kg  m_nominal_specify=off  m_nominal_value=1  m_nominal_unit=kg  T_specify=off  T_priority=None  T=308.15 K  T_nominal_specify=off  T_nominal_value=1  T_nominal_unit=K  Q_specify=off  Q_priority=None  Q=0 W  Q_nominal_specify=off  Q_nominal_value=1  Q_nominal_unit=W
  Token Rate : FromWorkspace  VariableName=tokenRateProfile  SampleTime=Ts  OutputAfterFinalValue=Holding final value
  Token to Utilization : Lookup_n-D  NumberOfTableDimensions=1  BreakpointsForDimension1=[0 1e-4 0.25 0.5 0.75 1.0]  Table=[0 0 0.25 0.5 0.75 1.0]  ExtrapMethod=Clip  InternalRulePriority=Speed  RndMeth=Simplest
  ~ : PMIOPort  Side=Left
  wires:
  Token Rate/1 -> Token to Utilization/1
  Token to Utilization/1 -> Gain1/1
  Gain1/1 -> Simulink-PS Converter/1
  connections:
  ~/RConn1 -- Load/LConn1
  Simulink-PS Converter/RConn1 -- PDU Racks/LConn2 -- PDU Racks/LConn1
  PDU Racks/RConn1 -- Efficiency Gain/LConn1
  Efficiency Gain/RConn1 -- THD/LConn1
  THD/RConn1 -- Load/LConn2
  THD/RConn2 -- Load/LConn3
  PDU Racks/LConn3 -- TermC_Ha/LConn1
  PDU Racks/RConn4 -- TermC_Hc/LConn1

== system UPSControl/Server Load/Signal Logging ==
  Meas : Inport
  Bus Selector : BusSelector  OutputSignals=activePower,reactivePower,Vdc,ILoad,IDCDC,voltage,Idc,IBatt,UPSBrK,rmsVoltage
  Terminator{,1..9} (10 alike) : Terminator
  wires:
  Bus Selector/3 -> Terminator2/1  "<Vdc>"
  Bus Selector/7 -> Terminator4/1  "<Idc>"
  Bus Selector/8 -> Terminator3/1  "<IBatt>"
  Bus Selector/4 -> Terminator5/1  "<ILoad>"
  Bus Selector/6 -> Terminator6/1  "<voltage>"
  Bus Selector/5 -> Terminator7/1  "<IDCDC>"
  Meas/1 -> Bus Selector/1
  Bus Selector/1 -> Terminator/1  "<activePower>"
  Bus Selector/2 -> Terminator9/1  "<reactivePower>"
  Bus Selector/9 -> Terminator1/1  "<UPSBrK>"
  Bus Selector/10 -> Terminator8/1  "<rmsVoltage>"

== system UPSControl/Server Load/UPS Units ==
  iChrg : Inport
  Single UPS : Subsystem  VariantControl=upsConfig == 1
  Three UPS Parallel : Subsystem  VariantControl=upsConfig == 3
  GridSide : PMIOPort  Side=Left
  LoadSide : PMIOPort  Port=2  Side=Right
  Meas : Outport
  P : Outport  Port=2
  Q : Outport  Port=3
